simulink model "NetworkModelSimpleIntersectionRDD"  (R2018b)
settings: Solver=VariableStepAuto  StartTime=tStart  StopTime=tFinal  FixedStep=0.001  RelTol=1e-3
undefined symbols (not defined in the file or in its folder): Ax, Ay, Bx, By, ConflictDrone2andDrone4, Cpx, Cpy, Cvx, Cvy, theta2, theta4, VelocityStarX2, VelocityStarX4, VelocityStarY2, VelocityStarY4, X20, X40, Y20, Y40
libraries: simulink x4
settings Model: Creator=CowUser  LastModifiedBy=CowUser

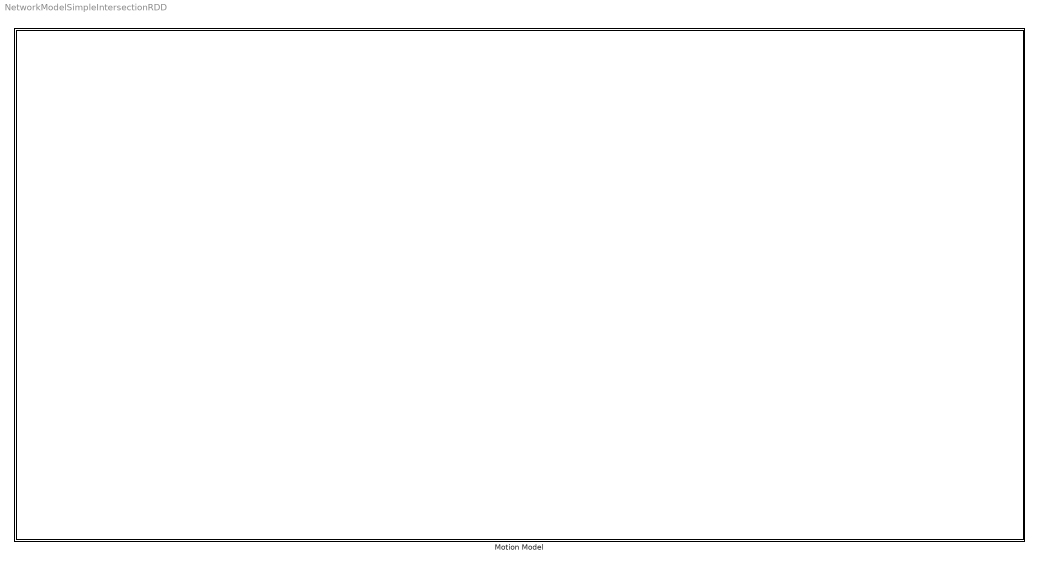
== system NetworkModelSimpleIntersectionRDD ==
  Motion Model : Subsystem

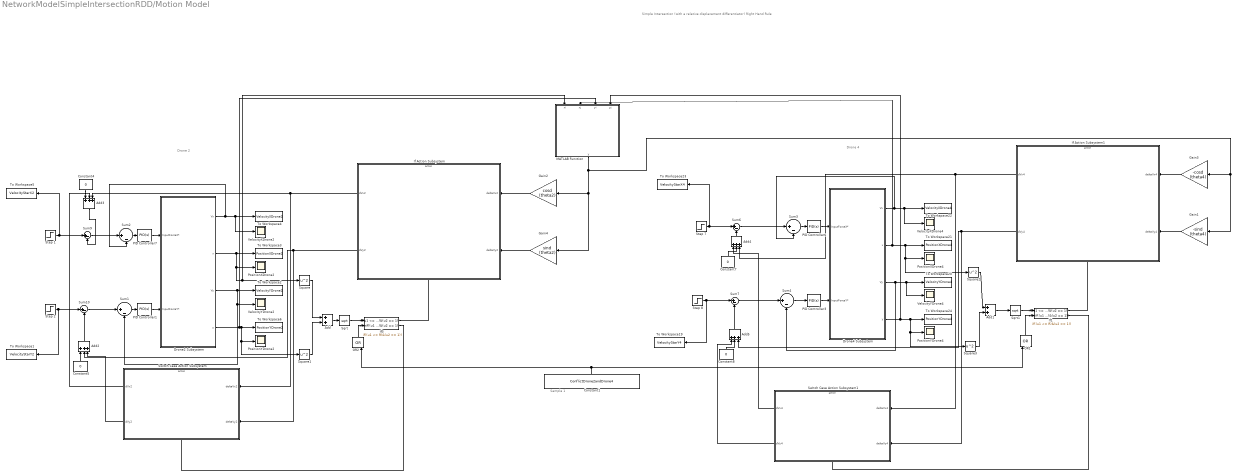
== system NetworkModelSimpleIntersectionRDD/Motion Model ==
  note: Sample 1
  note: Drone 4
  note: Drone 2
  note: Simple Intersection
      | (with a relative displacement differentiator)
      |
      | Right Hand Rule
  Add : Sum
  Add1 : Sum
  Add{2..5} (4 alike) : Sum  Inputs=+++
  Constant1 : Constant  Value=ConflictDrone2andDrone4
  Constant{4..5,7..8} (4 alike) : Constant  Value=0
  "Drone2 Subsystem " : Subsystem
  "Drone4 Subsystem " : Subsystem
  Gain1 : Gain  Gain=-sind (theta4)
  Gain2 : Gain  Gain=cosd (theta2)
  Gain3 : Gain  Gain=-cosd (theta4)
  Gain4 : Gain  Gain=sind (theta2)
  If Action Subsystem : Subsystem  TreatAsAtomicUnit=on
  If Action Subsystem1 : Subsystem  TreatAsAtomicUnit=on
  If1 : If  NumInputs=2  IfExpression=(u1 <= R)&(u2 == 1)  ElseIfExpressions=(u1 > R)&(u2 == 1)  ShowElse=off
  If3 : If  NumInputs=2  IfExpression=(u1 <= R)&(u2 == 1)  ElseIfExpressions=(u1 > R)&(u2 == 1)  ShowElse=off
  MATLAB Function : MATLAB Function  TreatAsAtomicUnit=on
  OR1 : Logic  Operator=OR  Inputs=3  IconShape=distinctive  AllPortsSameDT=off  OutDataTypeStr='double'
  OR2 : Logic  Operator=OR  Inputs=3  IconShape=distinctive  AllPortsSameDT=off  OutDataTypeStr='double'
  PID Controller{1,3,6..7} (4 alike) : simulink/Continuous/PID Controller  Controller=PID  Form=Parallel  TimeDomain=Continuous-time  SampleTime=-1  IntegratorMethod=Forward Euler  FilterMethod=Forward Euler  ControllerParametersSource=internal  P=1.97139727738968e-05  I=1.5233344900537e-08  D=0.00566857635684116  UseFilter=on  N=15.1370363747334  TunerSelectOption=Transfer Function Based (PID Tuner App)  InitialConditionSource=internal  InitialConditionForIntegrator=0  InitialConditionForFilter=0  DifferentiatorICPrevScaledInput=0  ExternalReset=none  TrackingMode=off  Kt=1  LimitOutput=off  UpperSaturationLimit=inf  LowerSaturationLimit=-inf  LinearizeAsGain=on  AntiWindupMode=none  Kb=1  POutMin=[]  POutMax=[]  IOutMin=[]  IOutMax=[]  DOutMin=[]  DOutMax=[]  NOutMin=[]  NOutMax=[]  SumOutMin=[]  SumOutMax=[]  SaturationOutMin=[]  SaturationOutMax=[]  PParamMin=[]  PParamMax=[]  IParamMin=[]  IParamMax=[]  DParamMin=[]  DParamMax=[]  NParamMin=[]  NParamMax=[]  KbParamMin=[]  KbParamMax=[]  KtParamMin=[]  KtParamMax=[]  KbOutMin=[]  KbOutMax=[]  KtOutMin=[]  KtOutMax=[]  IntegratorOutMin=[]  IntegratorOutMax=[]  FilterOutMin=[]  FilterOutMax=[]  SumI1OutMin=[]  SumI1OutMax=[]  SumI2OutMin=[]  SumI2OutMax=[]  SumI3OutMin=[]  SumI3OutMax=[]  SumI4OutMin=[]  SumI4OutMax=[]  SumDOutMin=[]  SumDOutMax=[]  DifferentiatorOutMin=[]  DifferentiatorOutMax=[]  FilterDiffOutCoefMin=[]  FilterDiffOutCoefMax=[]  ReciprocalOutMin=[]  ReciprocalOutMax=[]  SumDenOutMin=[]  SumDenOutMax=[]  SumNumOutMin=[]  SumNumOutMax=[]  DivideOutMin=[]  DivideOutMax=[]  IntegratorContinuousStateAttributes=''  IntegratorStateMustResolveToSignalObject=off  IntegratorRTWStateStorageClass=Auto  FilterContinuousStateAttributes=''  FilterStateMustResolveToSignalObject=off  FilterRTWStateStorageClass=Auto  ParallelPVariant=InternalParameters  IdealPVariant=Disabled  IVariant=InternalParameters  DVariant=InternalParameters  IntegratorVariant=Continuous  SatVariant=Disabled  AWVariant=Passthrough  PCopyVariant=Disabled  TRVariant=Disabled  FdbkBlocksVariant=Forward  IdealPFdbkVariant=Disabled  SatFdbkVariant=Disabled  DerivativeFilterVariant=ContFilter  NVariant=InternalParameters  NCopyVariant=Disabled  FilterICVariant=InternalICsFilter  IntegratorICVariant=InternalICs  ExternalResetVariant=Disabled  TRSumVariant=Passthrough  SumFdbkVariant=Disabled  SumVariant=Sum_PID
  PositionXDrone2 : Scope
  PositionXDrone4 : Scope
  PositionYDrone2 : Scope
  PositionYDrone4 : Scope
  Sqrt : Sqrt  SaturateOnIntegerOverflow=on
  Sqrt1 : Sqrt  SaturateOnIntegerOverflow=on
  Square{,1..3} (4 alike) : Math  Operator=square  SaturateOnIntegerOverflow=on
  Step 1 : Step  Time=0  After=VelocityStarX2  SampleTime=0
  Step 2 : Step  Time=0  After=VelocityStarY2  SampleTime=0
  Step 7 : Step  Time=0  After=VelocityStarX4  SampleTime=0
  Step 8 : Step  Time=0  After=VelocityStarY4  SampleTime=0
  Sum{1..4,6..7,9..10} (8 alike) : Sum  Inputs=|+-
  Switch Case Action Subsystem : Subsystem  TreatAsAtomicUnit=on
  Switch Case Action Subsystem1 : Subsystem  TreatAsAtomicUnit=on
  To Workspace1 : ToWorkspace  VariableName=VelocityStarY2  SampleTime=-1
  To Workspace19 : ToWorkspace  VariableName=VelocityStarY4  SampleTime=-1
  To Workspace2 : ToWorkspace  VariableName=VelocityYDrone2  SampleTime=-1
  To Workspace20 : ToWorkspace  VariableName=VelocityYDrone4  SampleTime=-1
  To Workspace21 : ToWorkspace  VariableName=PositionXDrone4  SampleTime=-1
  To Workspace22 : ToWorkspace  VariableName=VelocityXDrone4  SampleTime=-1
  To Workspace23 : ToWorkspace  VariableName=VelocityStarX4  SampleTime=-1
  To Workspace24 : ToWorkspace  VariableName=PositionYDrone4  SampleTime=-1
  To Workspace3 : ToWorkspace  VariableName=PositionXDrone2  SampleTime=-1
  To Workspace4 : ToWorkspace  VariableName=VelocityXDrone2  SampleTime=-1
  To Workspace5 : ToWorkspace  VariableName=VelocityStarX2  SampleTime=-1
  To Workspace6 : ToWorkspace  VariableName=PositionYDrone2  SampleTime=-1
  VelocityXDrone2 : Scope
  VelocityXDrone4 : Scope
  VelocityYDrone2 : Scope
  VelocityYDrone4 : Scope
  wires:
  If Action Subsystem1/2(dVy4) -> Switch Case Action Subsystem1/2(deltaVy4), Add5/3
  Constant8/1 -> Add5/2
  Constant4/1 -> Add3/2
  If Action Subsystem1/1(dVx4) -> Switch Case Action Subsystem1/1(deltaVx4), Add4/3
  "Drone2 Subsystem "/3(Vy) -> Sum1/2, VelocityYDrone2/1, To Workspace2/1
  Sum3/1 -> PID Controller6/1
  "Drone4 Subsystem "/1(Vx) -> Sum3/2, To Workspace22/1, VelocityXDrone4/1
  If Action Subsystem/2(dVy2) -> Add2/2, Switch Case Action Subsystem/2(deltaVy2)
  Sqrt1/1 -> If1/1
  Constant1/1 -> OR2/3, OR1/1
  If3/1 -> If Action Subsystem/Action
  Gain2/1 -> If Action Subsystem/1(deltaVx2)
  Sum2/1 -> PID Controller7/1
  Step 2/1 -> Sum10/1, To Workspace1/1
  Step 8/1 -> To Workspace19/1, Sum7/1
  Sqrt/1 -> If3/1
  If Action Subsystem/1(dVx2) -> Switch Case Action Subsystem/1(deltaVx2), Add3/3
  Sum10/1 -> Sum1/1
  "Drone2 Subsystem "/1(Vx) -> Sum2/2, VelocityXDrone2/1, To Workspace4/1
  Square2/1 -> Add1/1
  PID Controller1/1 -> "Drone2 Subsystem "/2("InputForceY* ")
  Square1/1 -> Add/2
  Square/1 -> Add/1
  "Drone4 Subsystem "/4(y) -> Square3/1, PositionYDrone4/1, To Workspace24/1, MATLAB Function/4(yj)
  Add1/1 -> Sqrt1/1
  If1/2 -> Switch Case Action Subsystem1/Action
  Constant7/1 -> Add4/2
  Switch Case Action Subsystem1/2(dVy4) -> Add5/1
  OR2/1 -> If3/2
  MATLAB Function/1(y) -> Gain4/1, Gain2/1, Gain3/1, Gain1/1
  Step 7/1 -> Sum6/1, To Workspace23/1
  "Drone4 Subsystem "/2(x) -> MATLAB Function/2(xj), Square2/1, PositionXDrone4/1, To Workspace21/1
  Gain1/1 -> If Action Subsystem1/2(deltaVy4)
  Gain3/1 -> If Action Subsystem1/1(deltaVx4)
  Constant5/1 -> Add2/1
  Switch Case Action Subsystem/1(dVx2) -> Add3/1
  Step 1/1 -> Sum9/1, To Workspace5/1
  Add3/1 -> Sum9/2
  Gain4/1 -> If Action Subsystem/2(deltaVy2)
  PID Controller6/1 -> "Drone4 Subsystem "/1(InputForceX*)
  Sum7/1 -> Sum4/1
  Add/1 -> Sqrt/1
  Add2/1 -> Sum10/2
  Switch Case Action Subsystem/2(dVy2) -> Add2/3
  Sum9/1 -> Sum2/1
  "Drone4 Subsystem "/3(Vy) -> Sum4/2, VelocityYDrone4/1, To Workspace20/1
  PID Controller3/1 -> "Drone4 Subsystem "/2("InputForceY* ")
  Sum6/1 -> Sum3/1
  "Drone2 Subsystem "/4(y) -> To Workspace6/1, Square1/1, PositionYDrone2/1, MATLAB Function/3(yi)
  "Drone2 Subsystem "/2(x) -> MATLAB Function/1(xi), Square/1, PositionXDrone2/1, To Workspace3/1
  If3/2 -> Switch Case Action Subsystem/Action
  Add4/1 -> Sum6/2
  OR1/1 -> If1/2
  Add5/1 -> Sum7/2
  Sum4/1 -> PID Controller3/1
  Sum1/1 -> PID Controller1/1
  Switch Case Action Subsystem1/1(dVx4) -> Add4/1
  If1/1 -> If Action Subsystem1/Action
  PID Controller7/1 -> "Drone2 Subsystem "/1(InputForceX*)
  Square3/1 -> Add1/2

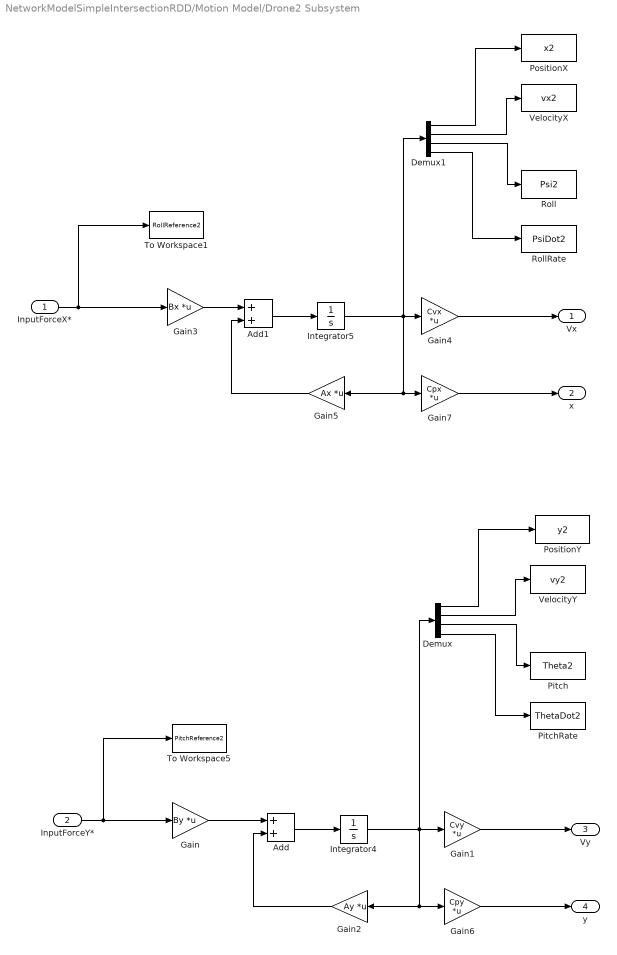
== system NetworkModelSimpleIntersectionRDD/Motion Model/Drone2 Subsystem  ==
  InputForceX* : Inport
  "InputForceY* " : Inport  Port=2
  Add : Sum
  Add1 : Sum
  Demux : Demux
  Demux1 : Demux
  Gain : Gain  Gain=By  Multiplication=Matrix(K*u)
  Gain1 : Gain  Gain=Cvy  Multiplication=Matrix(K*u)
  Gain2 : Gain  Gain=Ay  Multiplication=Matrix(K*u)
  Gain3 : Gain  Gain=Bx  Multiplication=Matrix(K*u)
  Gain4 : Gain  Gain=Cvx  Multiplication=Matrix(K*u)
  Gain5 : Gain  Gain=Ax  Multiplication=Matrix(K*u)
  Gain6 : Gain  Gain=Cpy  Multiplication=Matrix(K*u)
  Gain7 : Gain  Gain=Cpx  Multiplication=Matrix(K*u)
  Integrator4 : Integrator  InitialCondition=Y20
  Integrator5 : Integrator  InitialCondition=X20
  Pitch : ToWorkspace  VariableName=Theta2  SampleTime=-1
  PitchRate : ToWorkspace  VariableName=ThetaDot2  SampleTime=-1
  PositionX : ToWorkspace  VariableName=x2  SampleTime=-1
  PositionY : ToWorkspace  VariableName=y2  SampleTime=-1
  Roll : ToWorkspace  VariableName=Psi2  SampleTime=-1
  RollRate : ToWorkspace  VariableName=PsiDot2  SampleTime=-1
  To Workspace1 : ToWorkspace  VariableName=RollReference2  SampleTime=-1
  To Workspace5 : ToWorkspace  VariableName=PitchReference2  SampleTime=-1
  VelocityX : ToWorkspace  VariableName=vx2  SampleTime=-1
  VelocityY : ToWorkspace  VariableName=vy2  SampleTime=-1
  Vx : Outport
  x : Outport  Port=2
  Vy : Outport  Port=3
  y : Outport  Port=4
  wires:
  Demux/1 -> PositionY/1
  Demux1/2 -> VelocityX/1
  Demux1/4 -> RollRate/1
  Demux1/3 -> Roll/1
  Gain4/1 -> Vx/1
  "InputForceY* "/1 -> Gain/1, To Workspace5/1
  Gain/1 -> Add/1
  Demux/4 -> PitchRate/1
  Demux/3 -> Pitch/1
  Add/1 -> Integrator4/1
  Demux1/1 -> PositionX/1
  Gain1/1 -> Vy/1
  InputForceX*/1 -> Gain3/1, To Workspace1/1
  Gain7/1 -> x/1
  Integrator4/1 -> Gain6/1, Gain2/1, Demux/1, Gain1/1
  Demux/2 -> VelocityY/1
  Gain6/1 -> y/1
  Gain3/1 -> Add1/1
  Add1/1 -> Integrator5/1
  Gain2/1 -> Add/2
  Integrator5/1 -> Gain4/1, Gain5/1, Gain7/1, Demux1/1
  Gain5/1 -> Add1/2

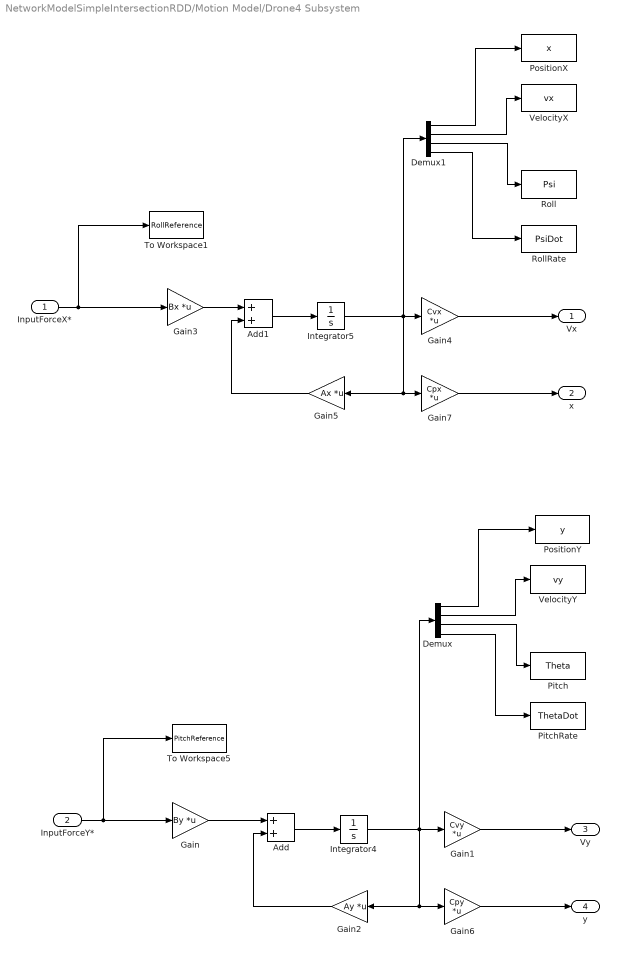
== system NetworkModelSimpleIntersectionRDD/Motion Model/Drone4 Subsystem  ==
  InputForceX* : Inport
  "InputForceY* " : Inport  Port=2
  Add : Sum
  Add1 : Sum
  Demux : Demux
  Demux1 : Demux
  Gain : Gain  Gain=By  Multiplication=Matrix(K*u)
  Gain1 : Gain  Gain=Cvy  Multiplication=Matrix(K*u)
  Gain2 : Gain  Gain=Ay  Multiplication=Matrix(K*u)
  Gain3 : Gain  Gain=Bx  Multiplication=Matrix(K*u)
  Gain4 : Gain  Gain=Cvx  Multiplication=Matrix(K*u)
  Gain5 : Gain  Gain=Ax  Multiplication=Matrix(K*u)
  Gain6 : Gain  Gain=Cpy  Multiplication=Matrix(K*u)
  Gain7 : Gain  Gain=Cpx  Multiplication=Matrix(K*u)
  Integrator4 : Integrator  InitialCondition=Y40
  Integrator5 : Integrator  InitialCondition=X40
  Pitch : ToWorkspace  VariableName=Theta  SampleTime=-1
  PitchRate : ToWorkspace  VariableName=ThetaDot  SampleTime=-1
  PositionX : ToWorkspace  VariableName=x  SampleTime=-1
  PositionY : ToWorkspace  VariableName=y  SampleTime=-1
  Roll : ToWorkspace  VariableName=Psi  SampleTime=-1
  RollRate : ToWorkspace  VariableName=PsiDot  SampleTime=-1
  To Workspace1 : ToWorkspace  VariableName=RollReference  SampleTime=-1
  To Workspace5 : ToWorkspace  VariableName=PitchReference  SampleTime=-1
  VelocityX : ToWorkspace  VariableName=vx  SampleTime=-1
  VelocityY : ToWorkspace  VariableName=vy  SampleTime=-1
  Vx : Outport
  x : Outport  Port=2
  Vy : Outport  Port=3
  y : Outport  Port=4
  wires:
  Gain4/1 -> Vx/1
  Demux/2 -> VelocityY/1
  Demux/4 -> PitchRate/1
  Gain3/1 -> Add1/1
  InputForceX*/1 -> Gain3/1, To Workspace1/1
  Gain2/1 -> Add/2
  Demux1/3 -> Roll/1
  Gain7/1 -> x/1
  Add1/1 -> Integrator5/1
  Demux/3 -> Pitch/1
  Gain5/1 -> Add1/2
  Gain6/1 -> y/1
  Integrator5/1 -> Gain4/1, Gain5/1, Gain7/1, Demux1/1
  Gain/1 -> Add/1
  Demux/1 -> PositionY/1
  Add/1 -> Integrator4/1
  Demux1/4 -> RollRate/1
  "InputForceY* "/1 -> Gain/1, To Workspace5/1
  Integrator4/1 -> Gain6/1, Gain2/1, Demux/1, Gain1/1
  Demux1/1 -> PositionX/1
  Demux1/2 -> VelocityX/1
  Gain1/1 -> Vy/1

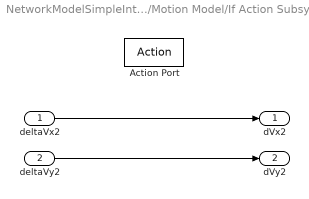
== system NetworkModelSimpleIntersectionRDD/Motion Model/If Action Subsystem ==
  deltaVx2 : Inport
  deltaVy2 : Inport  Port=2
  Action Port : ActionPort  ActionType=then
  dVx2 : Outport
  dVy2 : Outport  Port=2
  wires:
  deltaVx2/1 -> dVx2/1
  deltaVy2/1 -> dVy2/1

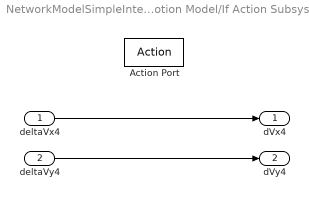
== system NetworkModelSimpleIntersectionRDD/Motion Model/If Action Subsystem1 ==
  deltaVx4 : Inport
  deltaVy4 : Inport  Port=2
  Action Port : ActionPort  ActionType=then
  dVx4 : Outport
  dVy4 : Outport  Port=2
  wires:
  deltaVx4/1 -> dVx4/1
  deltaVy4/1 -> dVy4/1

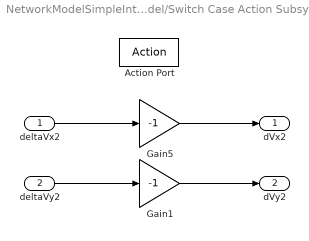
== system NetworkModelSimpleIntersectionRDD/Motion Model/Switch Case Action Subsystem ==
  deltaVx2 : Inport
  deltaVy2 : Inport  Port=2
  Action Port : ActionPort  ActionType=elseif
  Gain1 : Gain  Gain=-1
  Gain5 : Gain  Gain=-1
  dVx2 : Outport
  dVy2 : Outport  Port=2
  wires:
  deltaVy2/1 -> Gain1/1
  deltaVx2/1 -> Gain5/1
  Gain5/1 -> dVx2/1
  Gain1/1 -> dVy2/1

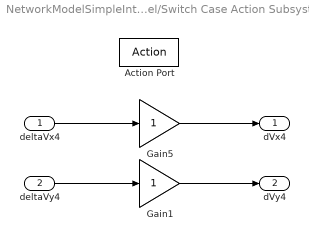
== system NetworkModelSimpleIntersectionRDD/Motion Model/Switch Case Action Subsystem1 ==
  deltaVx4 : Inport
  deltaVy4 : Inport  Port=2
  Action Port : ActionPort  ActionType=elseif
  Gain1 : Gain
  Gain5 : Gain
  dVx4 : Outport
  dVy4 : Outport  Port=2
  wires:
  deltaVy4/1 -> Gain1/1
  deltaVx4/1 -> Gain5/1
  Gain5/1 -> dVx4/1
  Gain1/1 -> dVy4/1

== matlab function NetworkModelSimpleIntersectionRDD/Motion Model/MATLAB Function ==
  data: xi input; y output; xj input; yi input; yj input
function y = VelocityChange(xi, xj, yi, yj)

Vmax = 0.2;
K = 1;
Vdiff = K/sqrt((xi - xj)^2 + (yi - yj)^2); 

if abs(Vdiff)>=Vmax/2
    Vdiff = Vmax/2;
end 

y = Vdiff;
